simulink model "prob9"  (R2020b)
settings: Solver=VariableStepAuto  StartTime=0.0  StopTime=1.2  RelTol=1e-3
model workspace (MAT data in the model file):
  Ke = 0.0275
  Kt = 0.0275
settings Model: Creator=nadee  LastModifiedBy=nadee

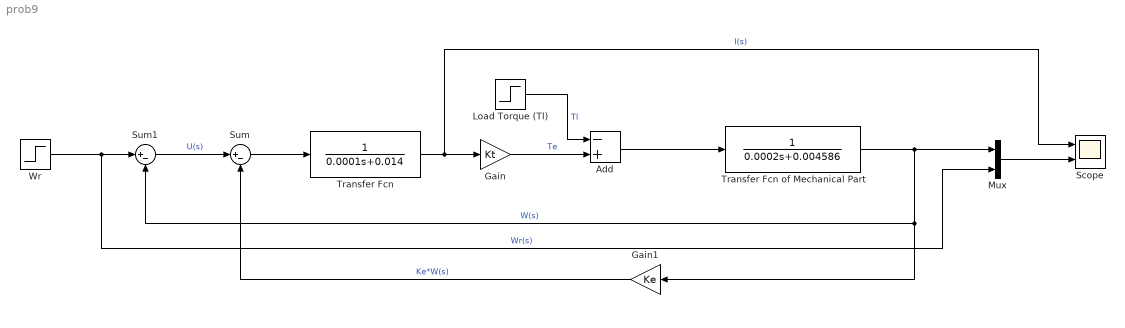
== system prob9 ==
  Add : Sum  Inputs=-+
  Gain : Gain  Gain=Kt
  Gain1 : Gain  Gain=Ke
  Load Torque (Tl) : Step  SampleTime=0
  Mux : Mux  Inputs=2
  Scope : Scope  NumInputPorts=2
  Sum : Sum  Inputs=|+-
  Sum1 : Sum  Inputs=|+-
  "Transfer Fcn " : TransferFcn  Denominator=[0.0001 0.014]
  Transfer Fcn of Mechanical Part : TransferFcn  Denominator=[0.0002 0.004586]
  Wr : Step  SampleTime=0
  wires:
  "Transfer Fcn "/1 -> Scope/1, Gain/1  "I(s)"
  Gain/1 -> Add/2  "Te"
  Load Torque (Tl)/1 -> Add/1  "Tl"
  Add/1 -> Transfer Fcn of Mechanical Part/1
  Transfer Fcn of Mechanical Part/1 -> Mux/1, Gain1/1, Sum1/2  "W(s)"
  Gain1/1 -> Sum/2  "Ke*W(s)"
  Sum/1 -> "Transfer Fcn "/1
  Sum1/1 -> Sum/1  "U(s)"
  Wr/1 -> Mux/2, Sum1/1  "Wr(s)"
  Mux/1 -> Scope/2
